simulink model "PV_model"  (R2024b)
settings: Solver=VariableStepAuto  StartTime=0.0  StopTime=200  RelTol=1e-3
values from neighbouring files (symbols this model uses):
  CellNum = 54    [Inititialisation.m]
  E_g = 1.1    [Inititialisation.m]
  G_ref = 1000    [Inititialisation.m]
  I_sc = 8.21    [Inititialisation.m]
  k_Boltz = 1.380649e-23    [Inititialisation.m]
  K_Isc = 0.0032    [Inititialisation.m]
  K_Vsc = -0.1230    (= -0.123)    [Inititialisation.m]
  n = 0.64611    [Inititialisation.m]
  Num_Paral = 1    [Inititialisation.m]
  NumSeries = 1    [Inititialisation.m]
  q = 1.60217663e-19    [Inititialisation.m]
  R_p = 65.4647    [Inititialisation.m]
  R_s = 0.47804    [Inititialisation.m]
  T_ref = 25+273.15    (= 298.15)    [Inititialisation.m]
  V_oc = 32.9    [Inititialisation.m]
undefined symbols (not defined in the file or in its folder): DataOutS4
libraries: fl_lib x4, nesl_utility x4, SignalEditorBlockLib x2
settings Model: Creator=Harrison  LastModifiedBy=Harrison
settings DebuggingCC: AlgebraicLoopMsg=none

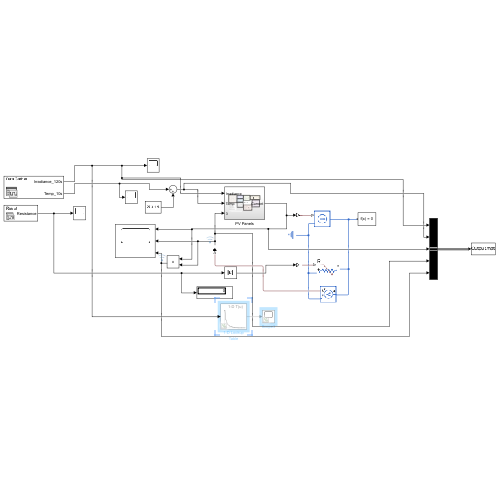
[thumbnail: Simulink's stored preview of the top-level diagram]
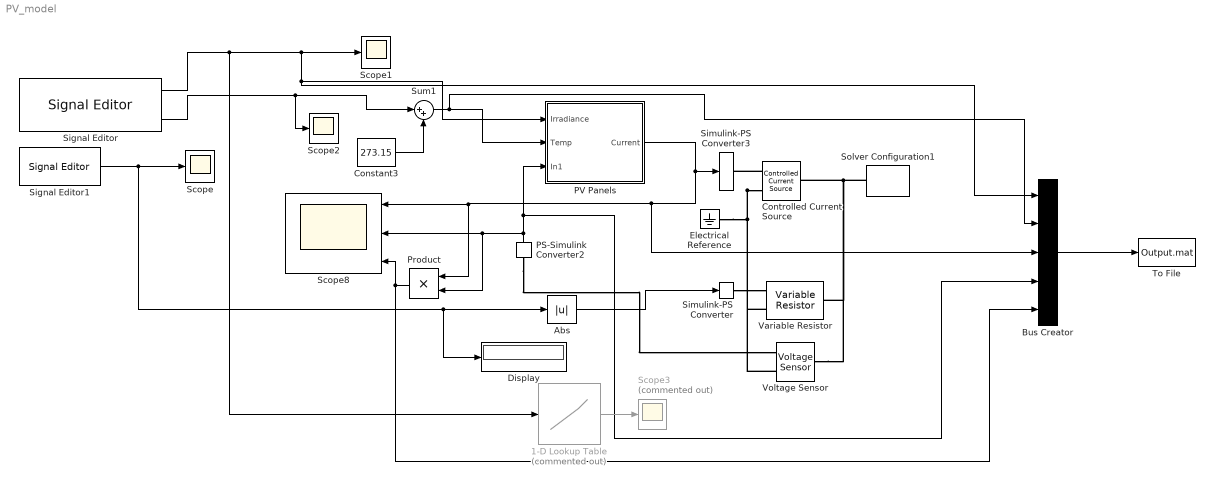
== system PV_model ==
  1-D Lookup Table : Lookup_n-D  Commented=on  NumberOfTableDimensions=1  BreakpointsForDimension1=[DataOutS4.Irrad]  Table=[DataOutS4.Resistance]  InternalRulePriority=Speed  RndMeth=Simplest
  Abs : Abs  SaturateOnIntegerOverflow=off
  Bus Creator : BusCreator  Inputs=5
  Constant3 : Constant  Value=273.15
  Controlled Current Source : fl_lib/Electrical/Electrical Sources/Controlled Current Source
  Display : Display
  Electrical Reference : fl_lib/Electrical/Electrical Elements/Electrical Reference
  PS-Simulink Converter2 : nesl_utility/PS-Simulink Converter  PhysicalDomain=network_engine_domain  SubClassName=ps_output  LeftPortType=input  RightPortType=output  PseudoPeriodic=off  Frequencies=[]  VectorFormat=inherit  Unit=inherit  AffineConversion=off
  PV Panels : Subsystem
  Product : Product
  Scope : Scope
  Scope1 : Scope
  Scope2 : Scope
  Scope3 : Scope  Commented=on
  Scope8 : Scope  NumInputPorts=3
  Signal Editor : SignalEditorBlockLib/Signal Editor  FileName=DataGather.mat  ActiveScenario=DataGather  ActiveSignal=Irradiance_120s  IsBus=off  OutputBusObjectStr=Bus: BusObject  SampleTime=0  Interpolate=off  ZeroCross=off  OutputAfterFinalValue=Setting to zero  Unit=inherit  PreserveSignalName=on  ApplySigPropsToAllScenarios=off  ApplySigPropsToAllSignals=off
  Signal Editor1 : SignalEditorBlockLib/Signal Editor  FileName=Resistance_DataGather.mat  ActiveScenario=Resist  ActiveSignal=Resistance  IsBus=off  OutputBusObjectStr=Bus: BusObject  SampleTime=0.01  ZeroCross=off  OutputAfterFinalValue=Setting to zero  Unit=inherit  PreserveSignalName=on  ApplySigPropsToAllScenarios=on  ApplySigPropsToAllSignals=off
  Simulink-PS Converter : nesl_utility/Simulink-PS Converter  PhysicalDomain=network_engine_domain  SubClassName=ps_input  LeftPortType=input  RightPortType=output  PseudoPeriodic=off  Frequencies=[]  NoiseDistribution=none  NoiseParameters=[]  Unit=1  AffineConversion=off  FilteringAndDerivatives=provide  SimscapeFilterOrder=1  InputFilterTimeConstant=0.001  UdotUserProvided=0
  Simulink-PS Converter3 : nesl_utility/Simulink-PS Converter  PhysicalDomain=network_engine_domain  SubClassName=ps_input  LeftPortType=input  RightPortType=output  PseudoPeriodic=off  Frequencies=[]  NoiseDistribution=none  NoiseParameters=[]  Unit=1  AffineConversion=off  FilteringAndDerivatives=provide  SimscapeFilterOrder=2  InputFilterTimeConstant=0.001  UdotUserProvided=0
  Solver Configuration1 : nesl_utility/Solver Configuration  PhysicalDomain=network_engine_domain  SubClassName=solver  LeftPortType=input  RightPortType=generic  Tones=[]  Harmonics=[]  SimulateNoise=off  Profile=off  UseLocalSampling=off  EnableSwitchedLinearOptims=on  FrequencyDomain=off  UseCCode=off  RelTol=0.001  AbsTol=0.001  MinStep=1e-09  ToWorkspace=off  RevertToSquareIcSolve=off  NumHomotopyIterations=100  PhasorMode=off  PhasorModeNumHarmonics=1  ConsistencySolver=NEWTON_XTOL_AFTER_FTOL  IndexReductionMethod=DerivativeReplacement  DoDC=off  ResidualTolerance=1e-09  ConsistencyTolSource=GLOBAL  ConsistencyAbsTol=0.001  ConsistencyRelTol=0.001  ConsistencyTolFactor=0.001  UseLocalSolver=off  LocalSolverChoice=NE_BACKWARD_EULER_ADVANCER  ResolveIndetEquations=on  FunctionEvalNumThread=1  LocalSolverSampleTime=0.001  DoFixedCost=off  MaxNonlinIter=3  MaxModeIter=2  ComputeImpulses=off  ImpulseIterations=2  LinearAlgebra=auto  LinearAlgebraNumThread=0  EquationFormulation=NE_TIME_EF  DelaysMemoryBudget=1024  AutomaticFiltering=on  FilteringTimeConstant=0.001  PartitionStorageMethod=AS_NEEDED  PartitionMemoryBudget=1024  PartitionMethod=ROBUST  MultibodyUseLocalSolver=off  MultibodyLocalSolverChoice=ODE1  MultibodyLocalSolverSampleTime=0.001
  Sum1 : Sum  Inputs=|++
  To File : ToFile  Filename=Output.mat  SaveFormat=Timeseries
      settings: Decimation=3
  Variable Resistor : fl_lib/Electrical/Electrical Elements/Variable Resistor  Rmin=0 Ohm  thermalEnable=false  thermal_mass=1 J/K  i_specify=off  i_priority=None  i=0 A  i_nominal_specify=off  i_nominal_value=1  i_nominal_unit=A  v_specify=off  v_priority=None  v=0 V  v_nominal_specify=off  v_nominal_value=1  v_nominal_unit=V  T_specify=off  T_priority=None  T=300 K  T_nominal_specify=off  T_nominal_value=1  T_nominal_unit=K
  Voltage Sensor : fl_lib/Electrical/Electrical Sensors/Voltage Sensor
  wires:
  Constant3/1 -> Sum1/2
  PS-Simulink Converter2/1 -> Bus Creator/4, PV Panels/3(In1), Product/2, Scope8/2
  Sum1/1 -> Bus Creator/2, PV Panels/2(Temp)
  PV Panels/1(Current) -> Bus Creator/3, Product/1, Scope8/1, Simulink-PS Converter3/1
  Product/1 -> Bus Creator/5, Scope8/3
  Signal Editor1/1 -> Display/1, Abs/1, Scope/1
  Signal Editor/2 -> Scope2/1, Sum1/1
  Signal Editor/1 -> 1-D Lookup Table/1, PV Panels/1(Irradiance), Bus Creator/1, Scope1/1
  Bus Creator/1 -> To File/1
  Abs/1 -> Simulink-PS Converter/1
  1-D Lookup Table/1 -> Scope3/1
  connections:
  Controlled Current Source/RConn2 -- Variable Resistor/LConn2 -- Voltage Sensor/RConn2 -- Electrical Reference/LConn1
  Solver Configuration1/RConn1 -- Voltage Sensor/LConn1 -- Variable Resistor/RConn1 -- Controlled Current Source/LConn1
  Controlled Current Source/RConn1 -- Simulink-PS Converter3/RConn1
  PS-Simulink Converter2/LConn1 -- Voltage Sensor/RConn1
  Simulink-PS Converter/RConn1 -- Variable Resistor/LConn1

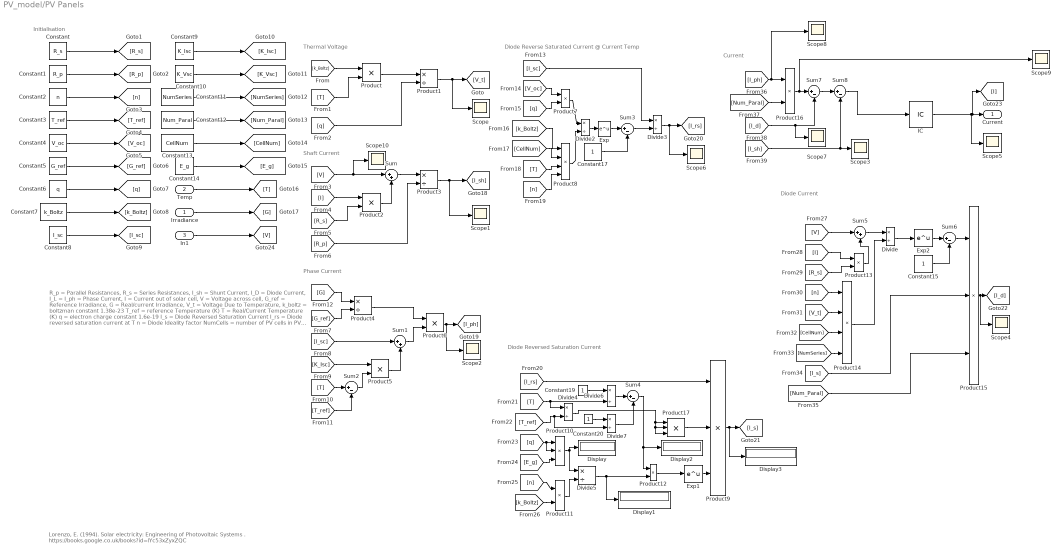
== system PV_model/PV Panels ==
  note: R_p = Parallel Resistances,
      | R_s = Series Resistances,
      | I_sh = Shunt Current,
      | I_D = Diode Current,
      | I_L = I_ph = Phase Current,
      | I = Current out of solar cell,
      | V = Voltage across cell,
      | G_ref = Reference Irradiance,
      | G = Real/current Irradiance,
      | V_t = Voltage Due to Temperature,
      | k_boltz = boltzman constant 1.38e-23
      | T_ref = reference Temperature (K)
      | T = Real/Current Temperature (K)
      | q = electron charge constant 1.6e-19
      | I_s = Diode Reversed Saturation Current
      | I_rs = Diode reversed saturation current at T
      | n = Diode Ideality factor
      | NumCells = number of PV cells in PV panel,
      | NumSeries = Number of PV panels in series,
      | Num_Paral = Number of PV panels in parallel,
      | E_g = Band gap energy of the cell, 1.12eV
  note: Lorenzo, E. (1994). Solar electricity: Engineering of Photovoltaic Systems . https://books.google.co.uk/books?id=lYc53xZyxZQC
  note: Initialisation
  note: Current
  note: Diode Current
  note: Diode Reversed Saturation Current
  note: Diode Reverse Saturated Current @ Current Temp
  note: Phase Current
  note: Shaft Current
  note: Thermal Voltage
  Irradiance : Inport
  Temp : Inport  Port=2
  In1 : Inport  Port=3
  Constant : Constant  Value=R_s
  Constant1 : Constant  Value=R_p
  Constant10 : Constant  Value=K_Vsc
  Constant11 : Constant  Value=NumSeries
  Constant12 : Constant  Value=Num_Paral
  Constant13 : Constant  Value=CellNum
  Constant14 : Constant  Value=E_g
  Constant{15,17,19..20} (4 alike) : Constant
  Constant2 : Constant  Value=n
  Constant3 : Constant  Value=T_ref
  Constant4 : Constant  Value=V_oc
  Constant5 : Constant  Value=G_ref
  Constant6 : Constant  Value=q
  Constant7 : Constant  Value=k_Boltz
  Constant8 : Constant  Value=I_sc
  Constant9 : Constant  Value=K_Isc
  Display{,1..3} (4 alike) : Display
  Divide{,2..7} (7 alike) : Product  Inputs=*/
  Exp : Math
  Exp1 : Math
  Exp2 : Math
  IC : InitialCondition  Value=0
  Product{,2,5..7,11..13,16} (9 alike) : Product
  Product1 : Product  Inputs=*/
  Product{9..10,15,17} (4 alike) : Product  Inputs=3
  Product14 : Product  Inputs=4
  Product3 : Product  Inputs=*/
  Product4 : Product  Inputs=*/
  Product8 : Product  Inputs=4
  Scope{,1..10} (11 alike) : Scope
  Sum : Sum  Inputs=|++
  Sum1 : Sum  Inputs=|++
  Sum{2..4,6..8} (6 alike) : Sum  Inputs=|+-
  Sum5 : Sum  Inputs=|++
  Current : Outport
  wires:
  [k_Boltz] -> Product/1
  [T] -> Product/2
  Product/1 -> Product1/1
  [q] -> Product1/2
  Product1/1 -> Scope/1, [V_t]
  Constant/1 -> [R_s]
  Constant1/1 -> [R_p]
  Constant2/1 -> [n]
  Constant3/1 -> [T_ref]
  Constant4/1 -> [V_oc]
  Constant5/1 -> [G_ref]
  Constant6/1 -> [q]
  Constant7/1 -> [k_Boltz]
  Constant8/1 -> [I_sc]
  Constant9/1 -> [K_Isc]
  Constant12/1 -> [Num_Paral]
  Constant10/1 -> [K_Vsc]
  Constant13/1 -> [CellNum]
  Constant11/1 -> [NumSeries]
  Constant14/1 -> [E_g]
  Temp/1 -> [T]
  Irradiance/1 -> [G]
  [R_s] -> Product2/2
  Product2/1 -> Sum/2
  Sum/1 -> Product3/1
  [R_p] -> Product3/2
  Product3/1 -> Scope1/1, [I_sh]
  [G] -> Product4/1
  [G_ref] -> Product4/2
  [I_sc] -> Sum1/1
  [K_Isc] -> Product5/1
  [T] -> Sum2/1
  [T_ref] -> Sum2/2
  Sum2/1 -> Product5/2
  Product5/1 -> Sum1/2
  Sum1/1 -> Product6/2
  Product4/1 -> Product6/1
  Product6/1 -> Scope2/1, [I_ph]
  [V_oc] -> Product7/1
  [q] -> Product7/2
  [k_Boltz] -> Product8/1
  [CellNum] -> Product8/2
  [T] -> Product8/3
  [n] -> Product8/4
  Product7/1 -> Divide2/1
  Product8/1 -> Divide2/2
  Divide2/1 -> Exp/1
  Exp/1 -> Sum3/1
  Constant17/1 -> Sum3/2
  Sum3/1 -> Divide3/2
  [I_sc] -> Divide3/1
  Divide3/1 -> Scope6/1, [I_rs]
  [T] -> Divide4/1, Divide6/2
  [T_ref] -> Divide7/2, Divide4/2
  [I_rs] -> Product9/1
  Exp1/1 -> Product9/3
  [q] -> Product10/2, Product10/1
  [E_g] -> Product10/3
  [n] -> Product11/1
  [k_Boltz] -> Product11/2
  Product10/1 -> Divide5/1, Display/1
  Product11/1 -> Divide5/2
  Constant19/1 -> Divide6/1
  Constant20/1 -> Divide7/1
  Divide6/1 -> Sum4/1
  Divide7/1 -> Sum4/2
  Divide5/1 -> Display1/1, Product12/2
  Sum4/1 -> Display2/1, Product12/1
  Product12/1 -> Exp1/1
  Product9/1 -> Display3/1, [I_s]
  [R_s] -> Product13/2
  Product13/1 -> Sum5/2
  Sum5/1 -> Divide/1
  [n] -> Product14/1
  [V_t] -> Product14/2
  [CellNum] -> Product14/3
  [NumSeries] -> Product14/4
  Product14/1 -> Divide/2
  Divide/1 -> Exp2/1
  Exp2/1 -> Sum6/1
  Constant15/1 -> Sum6/2
  Sum6/1 -> Product15/1
  [Num_Paral] -> Product15/3
  [I_s] -> Product15/2
  Product15/1 -> Scope4/1, [I_d]
  [I_ph] -> Scope8/1, Product16/1
  [Num_Paral] -> Product16/2
  Product16/1 -> Scope9/1, Sum7/1
  [I_d] -> Scope7/1, Sum7/2
  Sum7/1 -> Sum8/1
  [I_sh] -> Scope3/1, Sum8/2
  [V] -> Scope10/1, Sum/1
  [V] -> Sum5/1
  In1/1 -> [V]
  [I] -> Product2/1
  [I] -> Product13/1
  Sum8/1 -> IC/1
  IC/1 -> Scope5/1, [I], Current/1
  Product17/1 -> Product9/2
  Divide4/1 -> Product17/3, Product17/2, Product17/1
